simulink model "CTRL_LO_ST1_YAWTRQLGTDIST_test"  (R2023b)
settings: Solver=VariableStepAuto  StartTime=0.0  StopTime=10.0  RelTol=1e-3
libraries: CTRL_LO_ST1_YAWTRQLGTDIST x1
settings Model: Creator=blatak  LastModifiedBy=blatak

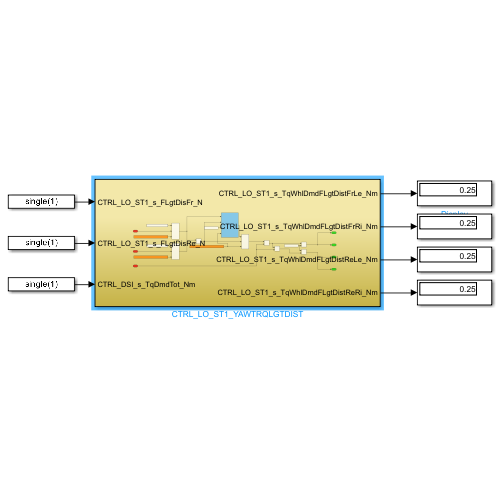
[thumbnail: Simulink's stored preview of the top-level diagram]
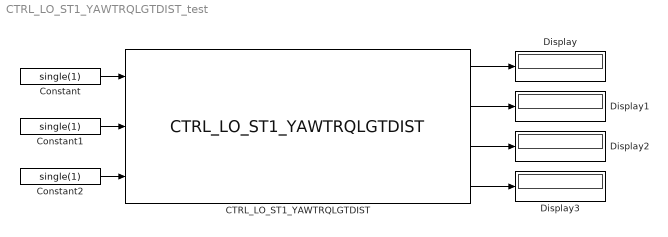
== system CTRL_LO_ST1_YAWTRQLGTDIST_test ==
  CTRL_LO_ST1_YAWTRQLGTDIST : CTRL_LO_ST1_YAWTRQLGTDIST/CTRL_LO_ST1_YAWTRQLGTDIST  SystemSampleTime=-1  VariantActivationTime=update diagram  AllowFlexibleInterface=on  Latency=0  AutoFrameSizeCalculation=off
  Constant : Constant  Value=single(1)
  Constant1 : Constant  Value=single(1)
  Constant2 : Constant  Value=single(1)
  Display{,1..3} (4 alike) : Display
  wires:
  Constant/1 -> CTRL_LO_ST1_YAWTRQLGTDIST/1
  Constant1/1 -> CTRL_LO_ST1_YAWTRQLGTDIST/2
  Constant2/1 -> CTRL_LO_ST1_YAWTRQLGTDIST/3
  CTRL_LO_ST1_YAWTRQLGTDIST/1 -> Display/1
  CTRL_LO_ST1_YAWTRQLGTDIST/2 -> Display1/1
  CTRL_LO_ST1_YAWTRQLGTDIST/3 -> Display2/1
  CTRL_LO_ST1_YAWTRQLGTDIST/4 -> Display3/1
